simulink model "ModelosMotores"  (R2020b)
settings: Solver=VariableStepAuto  StartTime=0.0  StopTime=20  MaxStep=0.01  RelTol=1e-3
undefined symbols (not defined in the file): B, Den, Go, Gpo, J, Ke, Kt, L, Num, Ra
settings Model: Creator=andre  LastModifiedBy=andre

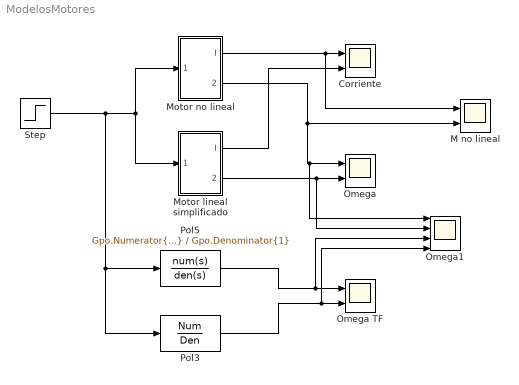
== system ModelosMotores ==
  Corriente : Scope  NumInputPorts=2
  M no lineal : Scope  NumInputPorts=2
  Motor lineal simplificado : Subsystem
  Motor no lineal : Subsystem
  Omega : Scope  NumInputPorts=2
  Omega TF : Scope  NumInputPorts=2
  Omega1 : Scope  NumInputPorts=4
  Pol3 : TransferFcn  Numerator=Num  Denominator=Den
  Pol5 : TransferFcn  Numerator=Gpo.Numerator{1}  Denominator=Gpo.Denominator{1}
  Step : Step  Time=0  SampleTime=0
  wires:
  Step/1 -> Pol3/1, Pol5/1, Motor lineal simplificado/1(In1), Motor no lineal/1(In1)
  Motor no lineal/1(I) -> M no lineal/1, Corriente/1
  Motor lineal simplificado/1(I) -> Corriente/2
  Motor no lineal/2(omega) -> M no lineal/2, Omega1/1, Omega/1
  Motor lineal simplificado/2(omega) -> Omega1/2, Omega/2
  Pol5/1 -> Omega1/3, Omega TF/1
  Pol3/1 -> Omega1/4, Omega TF/2

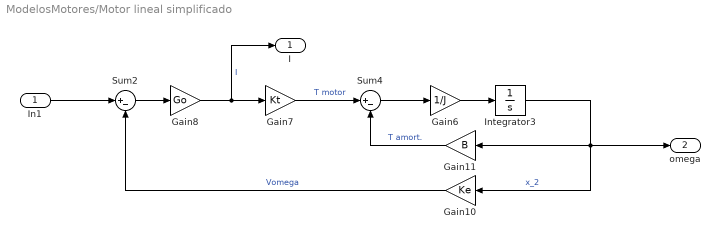
== system ModelosMotores/Motor lineal simplificado ==
  In1 : Inport
  Gain10 : Gain  Gain=Ke
  Gain11 : Gain  Gain=B
  Gain6 : Gain  Gain=1/J
  Gain7 : Gain  Gain=Kt
  Gain8 : Gain  Gain=Go
  Integrator3 : Integrator
  Sum2 : Sum  Inputs=|+-
  Sum4 : Sum  Inputs=|+-
  I : Outport
  omega : Outport  Port=2
  wires:
  Gain10/1 -> Sum2/2  "Vomega"
  Sum4/1 -> Gain6/1
  Integrator3/1 -> omega/1, Gain10/1, Gain11/1  "x_2"
  Gain11/1 -> Sum4/2  "T amort."
  Sum2/1 -> Gain8/1
  Gain7/1 -> Sum4/1  "T motor"
  Gain6/1 -> Integrator3/1
  Gain8/1 -> I/1, Gain7/1  "I"
  In1/1 -> Sum2/1

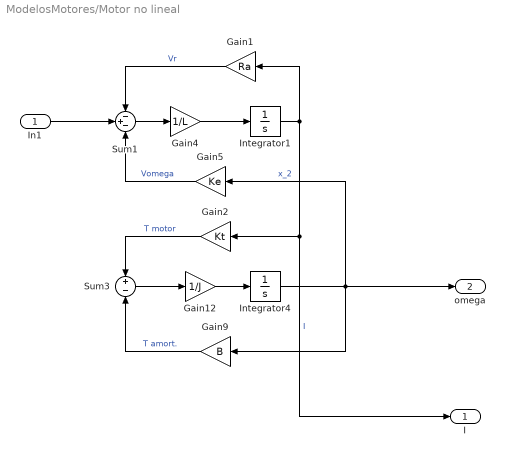
== system ModelosMotores/Motor no lineal ==
  In1 : Inport
  Gain1 : Gain  Gain=Ra
  Gain12 : Gain  Gain=1/J
  Gain2 : Gain  Gain=Kt
  Gain4 : Gain  Gain=1/L
  Gain5 : Gain  Gain=Ke
  Gain9 : Gain  Gain=B
  Integrator1 : Integrator
  Integrator4 : Integrator
  Sum1 : Sum  Inputs=-+-
  Sum3 : Sum  Inputs=+-
  I : Outport
  omega : Outport  Port=2
  wires:
  Integrator4/1 -> omega/1, Gain9/1, Gain5/1  "x_2"
  Integrator1/1 -> I/1, Gain2/1, Gain1/1  "I"
  Gain4/1 -> Integrator1/1
  Gain5/1 -> Sum1/3  "Vomega"
  Gain12/1 -> Integrator4/1
  Sum1/1 -> Gain4/1
  Sum3/1 -> Gain12/1
  Gain2/1 -> Sum3/1  "T motor"
  Gain1/1 -> Sum1/1  "Vr"
  Gain9/1 -> Sum3/2  "T amort."
  In1/1 -> Sum1/2
